simulink model "task_2_3"  (R2021b)
settings: Solver=VariableStepAuto  StartTime=0.0  StopTime=20  RelTol=1e-3
settings Model: Creator=osini  LastModifiedBy=osini

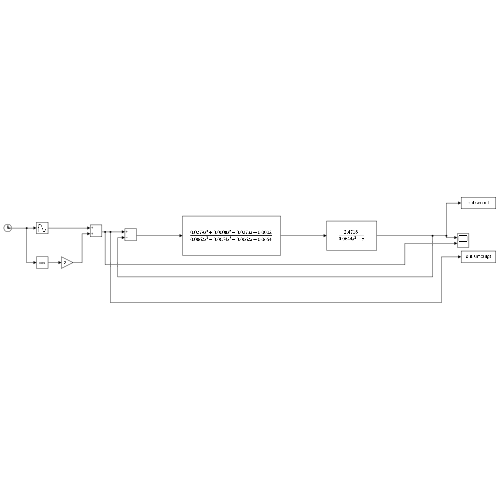
[thumbnail: Simulink's stored preview of the top-level diagram]
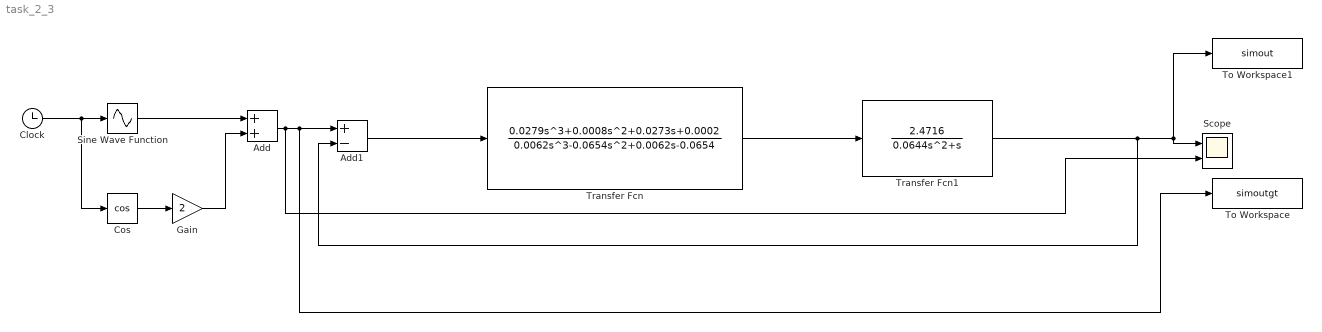
== system task_2_3 ==
  Add : Sum
  Add1 : Sum  Inputs=+-
  Clock : Clock
  Cos : Trigonometry  Operator=cos
  Gain : Gain  Gain=2
  Scope : Scope  NumInputPorts=2
  Sine Wave Function : Sin  TimeSource=Use external signal  Amplitude=3  Phase=1  SampleTime=0
  To Workspace : ToWorkspace  VariableName=simoutgt  SaveFormat=Timeseries  SampleTime=-1
  To Workspace1 : ToWorkspace  VariableName=simout  SaveFormat=Timeseries  SampleTime=-1
  Transfer Fcn : TransferFcn  Numerator="[0.0279    0.0008    0.0273    0.0002]"  Denominator="[0.0062   -0.0654    0.0062   -0.0654]"
  Transfer Fcn1 : TransferFcn  Numerator=[2.4716]  Denominator=[0.0644 1 0]
  wires:
  Clock/1 -> Cos/1, Sine Wave Function/1
  Cos/1 -> Gain/1
  Sine Wave Function/1 -> Add/1
  Gain/1 -> Add/2
  Transfer Fcn1/1 -> Add1/2, To Workspace1/1, Scope/1
  Add/1 -> Scope/2, To Workspace/1, Add1/1
  Transfer Fcn/1 -> Transfer Fcn1/1
  Add1/1 -> Transfer Fcn/1
